simulink library "mbed_lib"  (R2016b)
settings: Solver=ode45  StartTime=0.0  StopTime=10.0  RelTol=1e-3
undefined symbols (not defined in the file): A, PortWidth
libraries: mbed_lib x1
settings Model: Creator=syoon  LastModifiedBy=oh
settings DataIOCC: LimitDataPoints=on  SaveFormat=Array
settings OptimizationCC: BlockReduction=off  BooleanDataType=off  LifeSpan=inf
settings DebuggingCC: SaveWithParameterizedLinksMsg=none  UnderspecifiedInitializationDetection=Classic  MergeDetectMultiDrivingBlocksExec=none  SignalResolutionControl=TryResolveAllWithWarning  StrictBusMsg=Warning  SFUnexpectedBacktrackingDiag=warning  SFNoUnconditionalDefaultTransitionDiag=warning  SFExecutionAtInitializationDiag=none
settings HardwareCC: ProdBitPerPointer=32  ProdBitPerSizeT=32  ProdBitPerPtrDiffT=32  ProdLargestAtomicFloat=None  ProdIntDivRoundTo=Undefined  ProdEndianess=Unspecified  ProdWordSize=32  ProdHWDeviceType=32-bit Generic  TargetUnknown=on
settings ModelReferenceCC: PropagateSignalLabelsOutOfModel=off
settings GRTTargetCC: TargetLangStandard=C89/C90 (ANSI)  GeneratePreprocessorConditionals=Disable all
settings ConfigComp: CovMetricSettings=dw  CovHtmlReporting=on  CovSaveCumulativeToWorkspaceVar=on  CovSaveSingleToWorkspaceVar=on  CovExternalEMLEnable=off  CovSFcnEnable=off

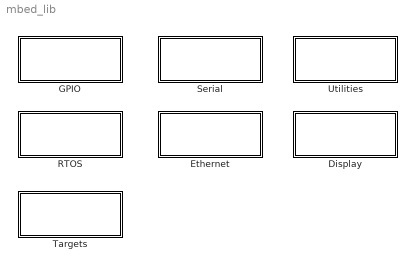
== system mbed_lib ==
  Display : Subsystem
      settings: OpenFcn=LCDScope
      mask Display: disp('Display')
  Ethernet : Subsystem
      settings: OpenFcn=mbed_ethernet
      mask Display: disp('Ethernet')
  GPIO : Subsystem
      mask Display: disp('GPIO')
  RTOS : Subsystem
      mask Display: disp('RTOS')
  Serial : Subsystem
      mask Display: disp('Serial')
  Targets : Subsystem
      settings: OpenFcn=mbed_targets
      mask Display: disp('Targets')
  Utilities : Subsystem
      mask Display: disp('Utilities')

== system mbed_lib/Display ==

== system mbed_lib/Ethernet ==

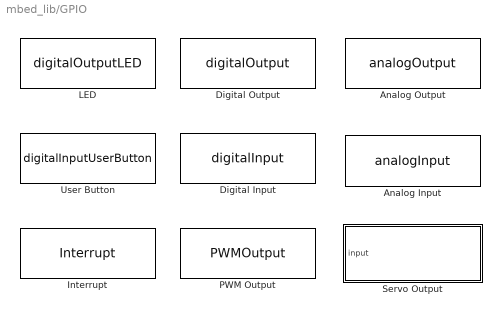
== system mbed_lib/GPIO ==
  Analog Input : S-Function  FunctionName=analogInput  Parameters=SampleTime, uint8(PortName), uint8(PinNumber)  SFunctionDeploymentMode=off  EnableBusSupport=off  mask(mbed Analog Input){PortName=A, PinNumber=0, SampleTime=-1}
      mask prompts: PortName "Port Name:"; PinNumber "Pin Number:"; SampleTime "Sample time (-1 for inherited):"
      mask help:
      | Reads the analog voltage input from the specified pin.
      |
      | The range of input on the pin is between 0 and Vref corresponding to a block output of 0 to 1.0f (in %) or 0 to 1024/4096/.. .
      mask Help: helpview(mbed_getHelpFile('analogInput'))
      mask TypeOptions PortName: A | B | C | D | E | F | G | H | I | J | K
      mask TypeOptions PinNumber: 0 | 1 | 2 | 3 | 4 | 5 | 6 | 7 | 8 | 9 | 10 | 11 | 12 | 13 | 14 | 15
      mask Display:
      | offset=0.0;
      | plot([0+offset:0.025:0.25+offset],0.3*sin(2*pi*[0:0.1:1])+0.5)
      | disp(['Pin ', PortName+64, '.', num2str(PinNumber-1)]);
      | port_label('output',1,'RAW');
      | port_label('output',2,'0-1.0f');
  Analog Output : S-Function  FunctionName=analogOutput  Parameters=SampleTime, uint8(PortName), uint8(PinNumber), uint8(Mode)  SFunctionDeploymentMode=off  EnableBusSupport=off  mask(mbed Analog Output){PortName=A, PinNumber=0, Mode=Double: 0 - 1.0f, SampleTime=-1}
      mask prompts: PortName "Port Name:"; PinNumber "Pin Number:"; Mode "Input data format"; SampleTime "Sample time (-1 for inherited):"
      mask help:
      | Writes an analog voltage output to the specified pin using the integrated DAC.
      |
      | The input to this block is a float between 0 and 1.0 (in %) or an integer between 0 and 1024/4096/.. corresponding to an output voltage between 0 to Vref.
      mask Help: helpview(mbed_getHelpFile('analogOutput'))
      mask TypeOptions PortName: A | B | C | D | E | F | G | H | I | J | K
      mask TypeOptions PinNumber: 0 | 1 | 2 | 3 | 4 | 5 | 6 | 7 | 8 | 9 | 10 | 11 | 12 | 13 | 14 | 15
      mask TypeOptions Mode: Uint16: RAW (0x0YYY) | Double: 0 - 1.0f
      mask Display:
      | offset=0.7;
      | plot([0+offset:0.025:0.25+offset],0.3*sin(2*pi*[0:0.1:1])+0.5)
      | disp(['Pin ', PortName+64, '.', num2str(PinNumber-1)]);
      | p={'RAW'; '0-1.0f'};
      | port_label('input',1,p{Mode});
  Digital Input : S-Function  FunctionName=digitalInput  Parameters=SampleTime, uint8(PortName), uint8(PinNumber), uint8(InputMode)  SFunctionDeploymentMode=off  EnableBusSupport=off  mask(mbed Digital Input){PortName=A, PinNumber=0, InputMode=PullDefault, SampleTime=-1}
      mask prompts: PortName "Port Name"; PinNumber "Pin Number:"; InputMode "Input Mode"; SampleTime "Sample time (-1 for inherited):"
      mask help:
      | Reads the digital value from the specified pin.
      |
      | The block outputs 1 for high and 0 for low.
      mask Help: helpview(mbed_getHelpFile('digitalInput'))
      mask TypeOptions PortName: A | B | C | D | E | F | G | H | I | J | K
      mask TypeOptions PinNumber: 0 | 1 | 2 | 3 | 4 | 5 | 6 | 7 | 8 | 9 | 10 | 11 | 12 | 13 | 14 | 15
      mask TypeOptions InputMode: PullDefault | PullUp | PullDown | PullNone
      mask Display:
      | plot([0 0.15 0.15 0.35 0.35 0.5],[0.3 0.3 0.7 0.7 0.3 0.3])
      | port_label('output',1,['Pin ', PortName+64, '.', num2str(PinNumber-1)]);
  Digital Output : S-Function  FunctionName=digitalOutput  Parameters=SampleTime, uint8(PortName), uint8(PinNumber), uint8(OutputMode)  SFunctionDeploymentMode=off  EnableBusSupport=off  mask(mbed Digital Output){PortName=A, PinNumber=0, OutputMode=PullDefault, SampleTime=-1}
      mask prompts: PortName "Port Name:"; PinNumber "Pin Number:"; OutputMode "Output Mode"; SampleTime "Sample time (-1 for inherited):"
      mask help:
      | Sends the digital value to the specified port.pin.
      |
      | The pin behaviour (pullup, pulldown, opendrain, ...) can be configured.
      |
      | An input of 1 sets the pin high and 0 sets the pin low.
      mask Help: helpview(mbed_getHelpFile('digitalOutput'))
      mask TypeOptions PortName: A | B | C | D | E | F | G | H | I | J | K
      mask TypeOptions PinNumber: 0 | 1 | 2 | 3 | 4 | 5 | 6 | 7 | 8 | 9 | 10 | 11 | 12 | 13 | 14 | 15
      mask TypeOptions OutputMode: PullDefault | PullUp | PullDown | PullNone | Repeater | OpenDrain
      mask Display:
      | plot([0.5 0.65 0.65 0.85 0.85 1],[0.3 0.3 0.7 0.7 0.3 0.3])
      | port_label('input',1,['Pin ', PortName+64, '.', num2str(PinNumber-1)]);
  Interrupt : S-Function  FunctionName=Interrupt  Parameters=uint8(PortName), uint8(PinNumber), uint8(Interrupt)  SFunctionDeploymentMode=off  EnableBusSupport=off  mask(mbed Interrupt Pin){PortName=A, PinNumber=0, Interrupt=Rise}
      mask prompts: PortName "Port Name"; PinNumber "Pin Name"
      mask help:
      | Defines the specified pin as an Interrupt pin. The interrupt can be generated by a rising, a falling or by both edges.
      |
      | A function-call subsystem can be connected with the output.
      mask Help: helpview(mbed_getHelpFile('Interrupt'))
      mask TypeOptions PortName: A | B | C | D | E | F | G | H | I | J | K
      mask TypeOptions PinNumber: 0 | 1 | 2 | 3 | 4 | 5 | 6 | 7 | 8 | 9 | 10 | 11 | 12 | 13 | 14 | 15
      mask TypeOptions Interrupt: None | Rise | Fall | Both
      mask Display:
      | p={'None'; 'Rise'; 'Fall'; 'Both'};
      | disp(['Interrupt: ' p{Interrupt} '          ']);
      | port_label('output',1,['Pin ', PortName+64, '.', num2str(PinNumber-1)]);
  LED : S-Function  FunctionName=digitalOutputLED  Parameters=SampleTime, uint8(nLED)  SFunctionDeploymentMode=off  EnableBusSupport=off  mask(mbed Digital Output LED){nLED=1, SampleTime=-1}
      mask prompts: nLED "LED Number:"; SampleTime "Sample time (-1 for inherited):"
      mask help:
      | Sends the digital value to the specified LED.
      |
      | An input of 1 sets the pin high and 0 sets the pin low.
      mask Help: helpview(mbed_getHelpFile('digitalOutputLED'))
      mask TypeOptions nLED: 1 | 2 | 3 | 4
      mask Display:
      | plot([0.5 0.65 0.65 0.85 0.85 0.85 1 0.5 0.65 0.65 0.85 0.85 0.85 1],[0.4 0.4 0.8 0.4 0.8 0.4 0.4 0.4 0.4 0.0 0.4 -0.0 0.4 0.4])
      | 
      | plot([0.75 0.8],[0.7 0.85])
      | plot([0.78 0.8],[0.825 0.85])
      | plot([0.79 0.8],[0.8 0.85])
      | 
      | plot([0.78 0.83],[0.7 0.85])
      | plot([0.815 0.83],[0.825 0.85])
      | plot([0.82 0.83],[0.8 0.85])
      | 
      | port_label('input',1,['LED' num2str(nLED)]);
  PWM Output : S-Function  FunctionName=PWMOutput  Parameters=SampleTime, uint8(PortName), uint8(PinNumber), uint32(Period)  SFunctionDeploymentMode=off  EnableBusSupport=off  mask(mbed PWM Output){PortName=A, PinNumber=0, Period=1000, SampleTime=-1}
      mask prompts: PortName "PWM Port:"; PinNumber "PWM Pin:"; Period "Period (µs):"; SampleTime "Sample time (-1 for inherited):"
      mask help:
      | Creates an pwm output signal on the specified pin using a configurable PWM period.
      |
      | The input to this block is a float between 0.0f and 1.0f corresponding to 0 to 100% pulsewidth.
      mask Help: helpview(mbed_getHelpFile('PWMOutput'))
      mask TypeOptions PortName: A | B | C | D | E | F | G | H | I | J | K
      mask TypeOptions PinNumber: 0 | 1 | 2 | 3 | 4 | 5 | 6 | 7 | 8 | 9 | 10 | 11 | 12 | 13 | 14 | 15
      mask Display:
      | plot([0.5 0.65 0.65 0.85 ],[0.3 0.3 0.7 0.7 ])
      | plot([0.8 0.8],[0.7 0.3])
      | plot([0.825 0.825],[0.7 0.3])
      | plot([0.85 0.85],[0.7 0.3])
      | plot([0.8 1],[0.3 0.3])
      | disp(['Pin ' PortName+64 '.' num2str(PinNumber-1)]);
      | port_label('input',1,'0-1.0f');
  Servo Output : Subsystem  mask(mbed Servo Output){PortName=A, PinNumber=0, PW_min=1, PW_max=2, SampleTime=-1}
      mask prompts: PortName "Port Name:"; PinNumber "Pin Number:"; PW_min "Pulse width min (ms)"; PW_max "max (ms)"; SampleTime "Sample time (-1 for inherited):"
      mask help:
      | Generates a PWM signal with a period of 20ms to control a standard RC-servo.
      | Minimal and maximal pulsewidth can be configured. Typical values are 1ms and 2ms.
      |
      | The input to this block is a float between 0.0f and 1.0f corresponding to a pulsewidth between the configured minimal to maximal values.
      mask Help: helpview(mbed_getHelpFile('Servo'))
      mask TypeOptions PortName: PWM Output/PortName
      mask TypeOptions PinNumber: PWM Output/PinNumber
      mask TypeOptions SampleTime: PWM Output/SampleTime
      mask Display:
      | disp('Servo Output\n');
      | disp(['\nPin ' PortName+64 '.' num2str(PinNumber-1) ]);
      | port_label('input',1,'0-1.0f');
  User Button : S-Function  FunctionName=digitalInputUserButton  Parameters=SampleTime  SFunctionDeploymentMode=off  EnableBusSupport=off  mask(mbed User Button){SampleTime=-1}
      mask prompts: SampleTime "Sample time (-1 for inherited):"
      mask help:
      | Reads the digital value from the User Button.
      |
      | The block outputs 1 for high and 0 for low. The
      mask Help: helpview(mbed_getHelpFile('digitalInputUserButton'))
      mask Display:
      | plot([0 0.15 0.35 ],[0.3 0.3 0.7])
      | plot([0.35 0.5],[0.3 0.3])
      | port_label('output',1,'UserButton');

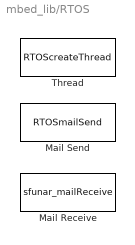
== system mbed_lib/RTOS ==
  Mail Receive : S-Function  FunctionName=sfunar_mailReceive  Parameters=MailNumber, uint32(DataType), uint32(NumElements)  SFunctionDeploymentMode=off  EnableBusSupport=off  mask{MailNumber=1, DataType=double, NumElements=1}
      mask prompts: MailNumber "Mail number"; DataType "Data type"; NumElements "Number of output elements"
      mask TypeOptions MailNumber: 1 | 2 | 3 | 4 | 5 | 6 | 7 | 8 | 9
      mask TypeOptions DataType: double | single | int8 | uint8 | int16 | uint16 | int32 | uint32
      mask Display:
      | disp(['Mail Receive\nInstance ' num2str(MailNumber)]);
      | port_label('output',1,'d');
      | port_label('output',2,'new');
  Mail Send : S-Function  FunctionName=RTOSmailSend  Parameters=MailNumber, DataType, uint32(NumElements), uint32(Depth)  SFunctionDeploymentMode=off  EnableBusSupport=off  mask(mbed RtosMail send){MailNumber=1, Depth=1, DataType=double, NumElements=1}
      mask prompts: MailNumber "Mail Instance Number"; Depth "Number of mails in queue"; DataType "Data type"; NumElements "Number of input elements"
      mask help:
      | Creates a rtos mailbox with the instance number 1...9.
      |
      | The maximal number of mails can be configured. Writing one mail more then this size will suspend the writing thread until the next mail is read.
      |
      | Each mail can contain the specified number of elements with the specified type.
      mask Help: helpview(mbed_getHelpFile('RTOSmailSend'))
      mask TypeOptions MailNumber: 1 | 2 | 3 | 4 | 5 | 6 | 7 | 8 | 9
      mask TypeOptions DataType: double | single | int8 | uint8 | int16 | uint16 | int32 | uint32
      mask Display:
      | disp(['Mail Send\nInstance ' num2str(MailNumber)]);
      | port_label('input',1,'d');
  Thread : S-Function  FunctionName=RTOScreateThread  Parameters=ThreadPriority, StackOption, uint32(StackSize), uint32(Timing)  SFunctionDeploymentMode=off  EnableBusSupport=off  mask(mbed create RTOS Thread){ThreadPriority=Normal, StackOption=Default, StackSize=0, Timing=0}
      mask prompts: ThreadPriority "Thread Priority"; StackOption "Stack size"; StackSize "Size: (bytes)"; Timing "Timing (ms)"
      mask help:
      | Creates a thread with the specified priority.
      |
      | Stack size can be DEFAULT_STACK_SIZE or have an individual value.
      |
      | When Timing equals 0, a Thread is created.
      | When Timing is greater then 0, a RtosTimer is created with this timing value (ms).
      | In both cases the function call subsystem is called in an endless loop (Thread) or a timed callback (RtosTimer).
      mask Help: helpview(mbed_getHelpFile('RTOScreateThread'))
      mask TypeOptions ThreadPriority: Idle | Low | Below Normal | Normal | Above Normal | High | Realtime
      mask TypeOptions StackOption: Default | User defined
      mask Display:
      | if Timing==0
      |   disp('create RtosThread');
      | else
      |   disp('create RtosTimer');
      | end

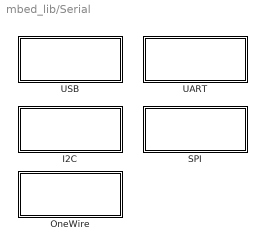
== system mbed_lib/Serial ==
  I2C : Subsystem
      mask Display: disp('I2C')
  OneWire : Subsystem
      mask Display: disp('OneWire')
  SPI : Subsystem
      mask Display: disp('SPI')
  UART : Subsystem
  USB : Subsystem

== system mbed_lib/Targets ==

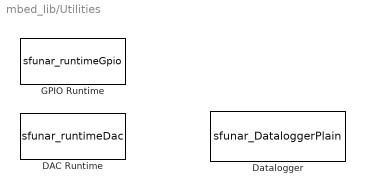
== system mbed_lib/Utilities ==
  DAC Runtime : S-Function  FunctionName=sfunar_runtimeDac  Parameters=SampleTime, PortName, PinNumber, DacValue  SFunctionDeploymentMode=off  EnableBusSupport=off  mask(DAC Runtime){PortName=A, PinNumber=0, DacValue=0, SampleTime=-1}
      mask prompts: PortName "Port Name"; PinNumber "Pin Number"; DacValue "DAC Value (0-1.0f)"; SampleTime "Sample time (-1 for inherited)"
      mask help:
      | Sets the DAC output to the configured value when entering the system that contains the block and resets the value after executing the systems code.
      | Can be used for time measurement of multiple subsystems, especially in multitasking models, using only one pin.
      | Setting each block to another DAC value and using an oscilloscope to differentiate between each subsystem.
      mask Help: helpview([mbed_getTargetRootPath '/doc/_build/htmlhelp/chapters/Dac_Runtime_en.html'])
      mask TypeOptions PortName: A | B | C | D | E | F | G | H | I | J
      mask TypeOptions PinNumber: 0 | 1 | 2 | 3 | 4 | 5 | 6 | 7 | 8 | 9 | 10 | 11 | 12 | 13 | 14 | 15
      mask Display:
      | disp('Runtime \nDAC Toggle\n');
      | disp(['\n\nPin ', PortName+64, '.', num2str(PinNumber-1) '  Value: ' num2str(DacValue) ]);
  Datalogger : S-Function  FunctionName=sfunar_DataloggerPlain  Parameters=TypeInputPorts, SampleTime, uint8(errEn), uint32(BufferSize)  SFunctionDeploymentMode=off  EnableBusSupport=off  mask(Creates a csv style string){TypeInputPorts={ 'uint8' 8 'int8' 4 'bool' 1 }, TypeOfInputs={'8*uint8' '4*int8' '1*bool'}, BufferSize=100, errEn=off, SampleTime=-1}
      mask prompts: TypeInputPorts "Type of Inputs"; TypeOfInputs "Type of Inputs"; BufferSize "Buffer Size"; errEn "Enable error output port"; SampleTime "Sample time (-1 for inherited):"
      mask help:
      | Type of Inputs:
      | List of 2-tuples
      |  1. item: Port width
      |  2. item: Port data type (single, double, int8, int16, int32, uint8, uint16, uint32, bool)
      |  e.g.: {'8*uint8' '4*int8' '1*bool'}
      |
      | Buffer Size:
      | Estimated maximal size of one data line.
      mask Callback TypeOfInputs:
      | cfg=eval(get_param(gcb,'TypeOfInputs'));
      | str={};
      | 
      | for i=1:size(cfg,2)
      |     res = strsplit(cfg{i}, '*');
      |     if isempty(str)
      |         str = strjoin({['''' res{2} ''''] res{1}});
      |     else
      |         str = strjoin({str ['''' res{2} ''''] res{1}});
      |     end
      | end
      | str = strjoin({'{' str '}'});
      | 
      | set_param(gcb,'TypeInputPorts', str);
      mask Display:
      | disp(['Datalogger']);
      | for i=1:2:size(TypeInputPorts,2)
      |     port_label('input',(i+1)/2, [TypeInputPorts{i} ':' num2str(TypeInputPorts{i+1})]);
      | end
      | port_label('output',1,'d');
      | port_label('output',2,'n');
      | if errEn
      |     port_label('output',3,'Error');
      | end
  GPIO Runtime : S-Function  FunctionName=sfunar_runtimeGpio  Parameters=SampleTime, PortName, PinNumber  SFunctionDeploymentMode=off  EnableBusSupport=off  mask(GPIO Runtime){PortName=A, PinNumber=0, SampleTime=-1}
      mask prompts: PortName "Port Name"; PinNumber "Pin Number"; SampleTime "Sample time (-1 for inherited)"
      mask help: Toggels a GPIO Pin so that the pulsewidth corresponds to the computational time of the containing subsystem.
      mask Help: helpview([mbed_getTargetRootPath '/doc/_build/htmlhelp/chapters/Gpio_Runtime_en.html'])
      mask TypeOptions PortName: A | B | C | D | E | F | G | H | I | J
      mask TypeOptions PinNumber: 0 | 1 | 2 | 3 | 4 | 5 | 6 | 7 | 8 | 9 | 10 | 11 | 12 | 13 | 14 | 15
      mask Display:
      | disp('Runtime \nGPIO Toggle\n');
      | disp(['\n\nPin ', PortName+64, '.', num2str(PinNumber-1)]);

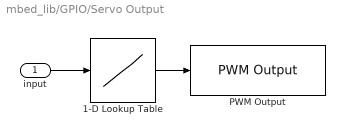
== system mbed_lib/GPIO/Servo Output ==
  input : Inport
  1-D Lookup Table : Lookup_n-D  NumberOfTableDimensions=1  BreakpointsForDimension1=[0 1]  Table=[PW_min PW_max]/20  ExtrapMethod=Clip  UseLastTableValue=on  InternalRulePriority=Speed  RndMeth=Simplest  InputSameDT=on
  PWM Output : mbed_lib/GPIO/PWM Output  PortName=A  PinNumber=0  Period=20000  SampleTime=SampleTime
  wires:
  input/1 -> 1-D Lookup Table/1
  1-D Lookup Table/1 -> PWM Output/1

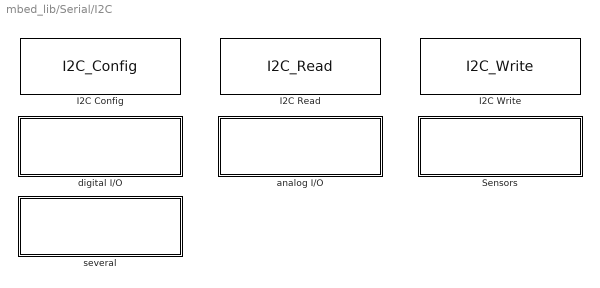
== system mbed_lib/Serial/I2C ==
  I2C Config : S-Function  Priority=0  FunctionName=I2C_Config  Parameters=uint8(SDAPortName), uint8(SDAPinNumber), uint8(SCLPortName), uint8(SCLPinNumber), uint32(Freq), uint8(I2CPort)  SFunctionDeploymentMode=off  EnableBusSupport=off  mask(I2C Configuration){I2CPort=1, Freq=100000, SDAPortName=B, SDAPinNumber=9, SCLPortName=B, SCLPinNumber=8}
      mask prompts: I2CPort "I2C Port"; Freq "Bus frequency: [Hz]"; SDAPortName "Port Name (SDA):"; SDAPinNumber "Pin Number:"; SCLPortName "Port Name (SCL):"; SCLPinNumber "Pin Number:"
      mask help:
      | This block sets up the I2C connection on the mbed board.
      |
      | To use several I2C busses at the mbed board, you can put several I2C Config blocks with different I2C Port numbers into the model. Each I2C Port number creates one instance of the mbed I2C class. The read and write blocks sending/receiving over the specific I2C bus have to use the same I2C Port number.
      mask Help: helpview(mbed_getHelpFile('I2CConfig'))
      mask TypeOptions I2CPort: 1 | 2 | 3
      mask TypeOptions SDAPortName: A | B | C | D | E | F
      mask TypeOptions SDAPinNumber: 0 | 1 | 2 | 3 | 4 | 5 | 6 | 7 | 8 | 9 | 10 | 11 | 12 | 13 | 14 | 15
      mask TypeOptions SCLPortName: A | B | C | D | E | F
      mask TypeOptions SCLPinNumber: 0 | 1 | 2 | 3 | 4 | 5 | 6 | 7 | 8 | 9 | 10 | 11 | 12 | 13 | 14 | 15
      mask Display:
      | disp(['I2C ' num2str(I2CPort) '\n\n']);
      | disp(['SDA: ' SDAPortName+64 '.' num2str(SDAPinNumber-1) ', SCL: ' SCLPortName+64, '.' num2str(SCLPinNumber-1)]);
      | disp(['\n\nFrequency: ' num2str(Freq) ' HZ']);
  I2C Read : S-Function  FunctionName=I2C_Read  Parameters=SampleTime, boolean(AddressFlag), uint8(SlaveAddress), boolean(ByteCountFlag), uint8(NumBytes), boolean(Repeated), uint8(I2cPort), boolean(AckOut)  SFunctionDeploymentMode=off  EnableBusSupport=off  mask(I2C Read){I2cPort=1, AddressFlag=off, SlaveAddress=0, ByteCountFlag=off, NumBytes=1, Repeated=off, AckOut=off, SampleTime=-1}
      mask prompts: I2cPort "I2C Port:"; AddressFlag "Enable address input port"; SlaveAddress "Slave address (8Bit):"; ByteCountFlag "Enable byte count input port"; NumBytes "Number of bytes to read:"; AckOut "Enable ack ouput port"; SampleTime "Sample time (-1 for inherited):"
      mask help: Performs a read operation from the device at the given i2c bus address.
      mask Help: helpview(mbed_getHelpFile('I2CRead'))
      mask TypeOptions I2cPort: 1 | 2 | 3
      mask Display:
      | disp(['I2C ' num2str(I2cPort) '\n']);
      | if AddressFlag == 0
      |     disp(['\nAddress: 0x' dec2hex(SlaveAddress)]);
      | else
      |    disp(['\nAddress: external']);
      |    port_label('input',1,'addr');
      | end
      | 
      | if ByteCountFlag == 1 && AddressFlag == 0
      |     port_label('input',1,'n');
      | elseif ByteCountFlag == 1 && AddressFlag == 1
      |     port_label('input',2,'n');
      | end
      | 
      | port_label('output',1,'d');
      | if AckOut == 1
      |     port_label('output',2,'ack');
      | end
  I2C Write : S-Function  FunctionName=I2C_Write  Parameters=SampleTime, boolean(AddressFlag), uint8(SlaveAddress), boolean(ByteCountFlag), boolean(Repeated), uint8(I2cPort), boolean(AckOut)  SFunctionDeploymentMode=off  EnableBusSupport=off  mask(I2C Write){I2cPort=1, AddressFlag=off, SlaveAddress=0, ByteCountFlag=off, Repeated=off, AckOut=off, SampleTime=-1}
      mask prompts: I2cPort "I2C Port:"; AddressFlag "Enable address input port"; SlaveAddress "Slave address (8Bit):"; ByteCountFlag "Enable byte count input port"; AckOut "Enable ack output port"; SampleTime "Sample time (-1 for inherited):"
      mask help: Performs a write operation to the device at the given i2c bus address.
      mask Help: helpview(mbed_getHelpFile('I2CWrite'))
      mask TypeOptions I2cPort: 1 | 2 | 3
      mask Display:
      | disp(['I2C ' num2str(I2cPort) '\n']);
      | 
      | port_label('input', 1, 'd');
      | 
      | if AddressFlag == 1
      |     disp(['\nAddress: external']);
      |     port_label('input', 2, 'addr');
      | else
      |     disp(['\nAddress: 0x' dec2hex(SlaveAddress)]);
      | end
      | 
      | if AddressFlag == 0 && ByteCountFlag == 1
      |     port_label('input', 2, 'n');
      | elseif AddressFlag == 1 && ByteCountFlag == 1
      |     port_label('input', 3, 'n');
      | end
      | 
      | if AckOut == 1
      |     port_label('output',1,'ack');
      | end
  Sensors : Subsystem
      settings: OpenFcn=mbed_i2c_sensors
  analog I/O : Subsystem
      settings: OpenFcn=mbed_i2c_analog_io
  digital I/O : Subsystem
      settings: OpenFcn=mbed_i2c_digital_io
  several : Subsystem
      settings: OpenFcn=mbed_i2c_several

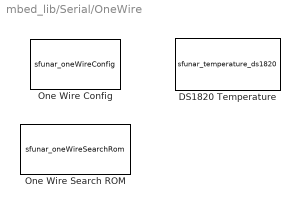
== system mbed_lib/Serial/OneWire ==
  DS1820 Temperature : S-Function  FunctionName=sfunar_temperature_ds1820  Parameters=OwBus, DeviceId, IDavail  SFunctionDeploymentMode=off  EnableBusSupport=off  mask(DS1820 Temperature){OwBus=1, DeviceId=[0 0 0 0 0 0]}
      mask prompts: OwBus "One Wire Bus"; DeviceId "Device ID (48 Bit)"
      mask help:
      | Reads the temperature measurement of a DS1820 (or DS18B20) One Wire temperature sensor.
      |
      | Output datatype:
      |     single
      mask init:
      | if (numel(DeviceId) == 0)
      |     IDavail = 0;
      |     DeviceId = 0;
      | else
      |     DeviceId = eval(DeviceId);
      |     if numel(DeviceId) ~= 6
      |         error('Device ID must contain 6 bytes');
      |     else
      |         IDavail = 1;
      |     end    
      | end
      mask Help: helpview([mbed_getTargetRootPath '/doc/_build/htmlhelp/sensor_actuator/DS1820_Temperature_en.html'])
      mask TypeOptions OwBus: 1 | 2 | 3 | 4 | 5 | 6 | 7 | 8 | 9
      mask Display:
      | disp(['DS1820 Temperature\n\n']);
      | disp(['\nOW Bus ' num2str(OwBus)]);
      | 
      | port_label('output',1,'°C');
  One Wire Config : S-Function  FunctionName=sfunar_oneWireConfig  Parameters=OwBus, OwPort, OwPin  SFunctionDeploymentMode=off  EnableBusSupport=off  mask(One Wire Config){OwBus=1, OwPort=A, OwPin=0}
      mask prompts: OwBus "OneWire Bus"; OwPort "OneWire Port:"; OwPin "Pin:"
      mask help: Configuration of a GPIO pin to be used as data line in a One Wire bus.
      mask Help: helpview([mbed_getTargetRootPath '/doc/_build/htmlhelp/mbed/one_wire_config_en.html'])
      mask TypeOptions OwBus: 1 | 2 | 3 | 4 | 5 | 6 | 7 | 8 | 9
      mask TypeOptions OwPort: A | B | C | D | E | F | G | H
      mask TypeOptions OwPin: 0 | 1 | 2 | 3 | 4 | 5 | 6 | 7 | 8 | 9 | 10 | 11 | 12 | 13 | 14 | 15
      mask Display:
      | disp('One Wire Config\n\n')
      | disp(['\nOW Bus ' num2str(OwBus)]);
      | disp(['\n\n\nPin: ' OwPort+64 '.' num2str(OwPin-1)]);
  One Wire Search ROM : S-Function  FunctionName=sfunar_oneWireSearchRom  Parameters=OwBus  SFunctionDeploymentMode=off  EnableBusSupport=off  mask{OwBus=1}
      mask prompts: OwBus "One Wire Bus"
      mask TypeOptions OwBus: 1 | 2 | 3 | 4 | 5 | 6 | 7 | 8 | 9
      mask Display:
      | disp('Search ROM\n\n')
      | disp(['\nOW Bus ' num2str(OwBus)]);
      | 
      | port_label('output',1,'ID');

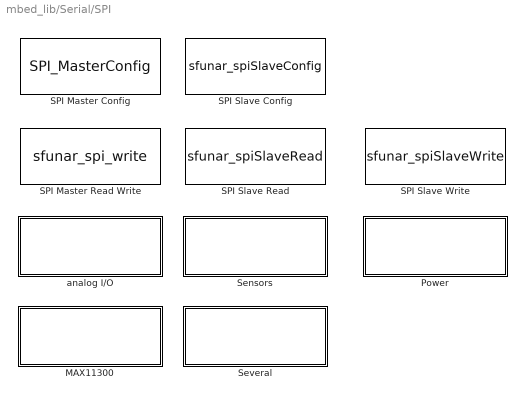
== system mbed_lib/Serial/SPI ==
  MAX11300 : Subsystem
      settings: OpenFcn=mbed_spi_max11300
  Power : Subsystem
      settings: OpenFcn=mbed_spi_power
  SPI Master Config : S-Function  Priority=0  FunctionName=SPI_MasterConfig  Parameters=uint8(MOSIPortName), uint8(MOSIPinNumber), uint8(MISOPortName), uint8(MISOPinNumber), uint8(SCLKPortName), uint8(SCLKPinNumber), uint32(Freq), uint8(Mode), uint8(Bits), uint8(SPIPort)  SFunctionDeploymentMode=off  EnableBusSupport=off  mask(SPI Configuration){SPIPort=1, Freq=100000, Mode=0, Bits=8, MOSIPortName=A, MOSIPinNumber=7, MISOPortName=A, MISOPinNumber=6, SCLKPortName=A, SCLKPinNumber=5}
      mask prompts: SPIPort "SPI Port"; Freq "Bus frequency: [Hz]"; MOSIPortName "MOSI: Port"; MOSIPinNumber "Pin"; MISOPortName "MISO: Port"; MISOPinNumber "Pin"; SCLKPortName "SCLK: Port"; SCLKPinNumber "Pin"
      mask help:
      | This block sets up the SPI connection on the mbed board. You must have one of these blocks in any model that ues SPI blocks.
      |
      | mode | POL PHA
      |  ------+--------
      |    0      |  0      0
      |    1      |  0      1
      |    2      |  1      0
      |    3      |  1      1
      mask Help: helpview([mbed_getTargetRootPath '/doc/_build/htmlhelp/chapters/Spi_Master_Config_en.html'])
      mask TypeOptions SPIPort: 1 | 2 | 3 | 4
      mask TypeOptions Mode: 0 | 1 | 2 | 3
      mask TypeOptions Bits: 4 | 5 | 6 | 7 | 8 | 9 | 10 | 11 | 12 | 13 | 14 | 15 | 16
      mask TypeOptions MOSIPortName: A | B | C | D | E | F | G | H | I | NC
      mask TypeOptions MOSIPinNumber: 0 | 1 | 2 | 3 | 4 | 5 | 6 | 7 | 8 | 9 | 10 | 11 | 12 | 13 | 14 | 15
      mask TypeOptions MISOPortName: A | B | C | D | E | F | G | H | I | NC
      mask TypeOptions MISOPinNumber: 0 | 1 | 2 | 3 | 4 | 5 | 6 | 7 | 8 | 9 | 10 | 11 | 12 | 13 | 14 | 15
      mask TypeOptions SCLKPortName: A | B | C | D | E | F | G | H | I
      mask TypeOptions SCLKPinNumber: 0 | 1 | 2 | 3 | 4 | 5 | 6 | 7 | 8 | 9 | 10 | 11 | 12 | 13 | 14 | 15
      mask Display:
      | disp(['SPI ' num2str(SPIPort) '\n\n\n']);
      | str1='';
      | if MOSIPortName==10
      |   str1 = 'NC';
      | else
      |   str1 = ['P' MOSIPortName+64 '.' num2str(MOSIPinNumber-1)];
      | end
      | str2='';
      | if MISOPortName==10
      |   str2 = 'NC';
      | else
      |   str2 = ['P' MISOPortName+64, '.' num2str(MISOPinNumber-1)];
      | end
      | disp(['\nMOSI: ' str1 ', MISO: ' str2 ' \n\n']);
      | disp(['\n\nSCK: P' SCLKPortName+64, '.' num2str(SCLKPinNumber-1) ' \n']);
      | disp(['\n\n\nFrequency: ' num2str(Freq) ' HZ']);
  SPI Master Read Write : S-Function  FunctionName=sfunar_spi_write  Parameters=SpiPort, CsPort, CsPin  SFunctionDeploymentMode=off  EnableBusSupport=off  mask(SPI Master Read Write){SpiPort=1, CsPort=A, CsPin=0}
      mask prompts: SpiPort "SPI Port"; CsPort "Chip Select Port"; CsPin "Pin"
      mask help: Perfoms a one byte write operation to the SPI bus and returns the received byte.
      mask Help: helpview([mbed_getTargetRootPath '/doc/_build/htmlhelp/chapters/Spi_Master_Read_Write_en.html'])
      mask TypeOptions SpiPort: 1 | 2 | 3 | 4
      mask TypeOptions CsPort: A | B | C | D | E | F | G | H
      mask TypeOptions CsPin: 0 | 1 | 2 | 3 | 4 | 5 | 6 | 7 | 8 | 9 | 10 | 11 | 12 | 13 | 14 | 15
      mask Display:
      | disp('SPI Master Read/Write\n\n');
      | disp(['SPI ' num2str(SpiPort)]);
      | 
      | disp(['\n\nChip Select: ' CsPort+64 '.' num2str(CsPin-1)]);
  SPI Slave Config : S-Function  FunctionName=sfunar_spiSlaveConfig  Parameters=BusSpeed, MosiPort, MosiPin, MisoPort, MisoPin, SckPort, SckPin, SselPort, SselPin  SFunctionDeploymentMode=off  EnableBusSupport=off  mask(SPI Slave Config){BusSpeed=100000, MosiPort=A, MosiPin=0, MisoPort=A, MisoPin=0, SckPort=A, SckPin=0, SselPort=A, SselPin=0}
      mask prompts: BusSpeed "Bus frequency: [Hz]"; MosiPort "MOSI: Port"; MosiPin "Pin"; MisoPort "MISO: Port"; MisoPin "Pin"; SckPort "SCK: Port"; SckPin "Pin"; SselPort "SSEL: Port"; SselPin "Pin"
      mask help: This block sets up the SPI connection on the mbed board to act as a slave device to an external master.
      mask Help: helpview([mbed_getTargetRootPath '/doc/_build/htmlhelp/chapters/Spi_Slave_Config_en.html'])
      mask TypeOptions MosiPort: A | B | C | D | E | F
      mask TypeOptions MosiPin: 0 | 1 | 2 | 3 | 4 | 5 | 6 | 7 | 8 | 9 | 10 | 11 | 12 | 13 | 14 | 15
      mask TypeOptions MisoPort: A | B | C | D | E | F
      mask TypeOptions MisoPin: 0 | 1 | 2 | 3 | 4 | 5 | 6 | 7 | 8 | 9 | 10 | 11 | 12 | 13 | 14 | 15
      mask TypeOptions SckPort: A | B | C | D | E | F
      mask TypeOptions SckPin: 0 | 1 | 2 | 3 | 4 | 5 | 6 | 7 | 8 | 9 | 10 | 11 | 12 | 13 | 14 | 15
      mask TypeOptions SselPort: A | B | C | D | E | F
      mask TypeOptions SselPin: 0 | 1 | 2 | 3 | 4 | 5 | 6 | 7 | 8 | 9 | 10 | 11 | 12 | 13 | 14 | 15
      mask Display:
      | disp(['Frequency: ' num2str(BusSpeed) ' HZ\n\n']);
      | disp(['\nMOSI: ' MosiPort+64 '.' num2str(MosiPin-1) ', MISO: ' MisoPort+64, '.' num2str(MisoPin-1) '\n']);
      | disp(['\n\n\nSCK: ' SckPort+64, '.' num2str(SckPin-1) ',SSEL: ' SselPort+64 '.' num2str(SselPin-1) '\n']);
  SPI Slave Read : S-Function  FunctionName=sfunar_spiSlaveRead  Parameters=SampleTime  SFunctionDeploymentMode=off  EnableBusSupport=off  mask(SPI Slave Read){SampleTime=-1}
      mask prompts: SampleTime "Sampel time: (-1 for inherited)"
      mask help: Reads the last received value from the spi input buffer.
      mask Help: helpview([mbed_getTargetRootPath '/doc/_build/htmlhelp/chapters/Spi_Slave_Read_en.html'])
      mask Display: disp('SPI Slave Read')
  SPI Slave Write : S-Function  FunctionName=sfunar_spiSlaveWrite  Parameters=SampleTime  SFunctionDeploymentMode=off  EnableBusSupport=off  mask(SPI Slave Write){SampleTime=-1}
      mask prompts: SampleTime "Sample time: (-1 for inherited)"
      mask help: This block puts one byte in the spi output buffer
      mask Help: helpview([mbed_getTargetRootPath '/doc/_build/htmlhelp/chapters/Spi_Slave_Write_en.html'])
      mask Display: disp('SPI Slave Write');
  Sensors : Subsystem
      settings: OpenFcn=mbed_spi_sensors
  Several : Subsystem
      settings: OpenFcn=mbed_spi_several
  analog I/O : Subsystem
      settings: OpenFcn=mbed_spi_analog_io

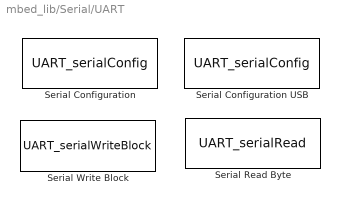
== system mbed_lib/Serial/UART ==
  Serial Configuration : S-Function  FunctionName=UART_serialConfig  Parameters=uint8(SerialPort), uint8(TXPort), uint8(TXPin), uint8(RXPort), uint8(RXPin), BaudRate  SFunctionDeploymentMode=off  EnableBusSupport=off  mask(mbed Serial Configuration){SerialPort=1, TXPort=A, TXPin=2, RXPort=A, RXPin=3, BaudRate=9600}
      mask prompts: SerialPort "Serial Port"; TXPort "Port Name (TX)"; TXPin "Pin Number (1-16):"; RXPort "Port Name (RX)"; RXPin "Pin Number (1-16):"; BaudRate "Baud Rate:"
      mask help:
      | This blocks sets up a serial connection on the mbed board. You must put at least one of these blocks into any model that ues the Serial Write or Serial Read blocks.
      |
      | To use several UARTS at the mbed board, you can put several Serial Config blocks with different Serial Port numbers into the model. Each Serial Port number creates one instance of the mbed Serial class. The read and write blocks sending/receiving over the specific UART have to use the same Serial Port number.
      |
      | Set the baud rate to match the device that you are communicating with. Standard rates include:300, 1200, 2400, 4800, 9600, 14400, 19200, 28800, 38400, 57600, or 115200.
      mask Help: helpview(mbed_getHelpFile('SerialUARTConfig'))
      mask TypeOptions SerialPort: 1 | 2 | 3 | 4 | 5
      mask TypeOptions TXPort: A | B | C | D | E | F
      mask TypeOptions TXPin: 0 | 1 | 2 | 3 | 4 | 5 | 6 | 7 | 8 | 9 | 10 | 11 | 12 | 13 | 14 | 15
      mask TypeOptions RXPort: A | B | C | D | E | F
      mask TypeOptions RXPin: 0 | 1 | 2 | 3 | 4 | 5 | 6 | 7 | 8 | 9 | 10 | 11 | 12 | 13 | 14 | 15
      mask Display: disp(['Serial config\nSerial' num2str(SerialPort) '\nTX ' TXPort+64 '.' num2str(TXPin-1) ', RX ' RXPort+64, '.' num2str(RXPin-1)]);
  Serial Configuration USB : S-Function  FunctionName=UART_serialConfig  Parameters=uint8(0), uint8(0), uint8(0), uint8(0), uint8(0), BaudRate  SFunctionDeploymentMode=off  EnableBusSupport=off  mask(mbed Serial Configuration){BaudRate=9600}
      mask prompts: BaudRate "Baud Rate:"
      mask help:
      | This blocks sets up the serial connection on the mbed board. You must have one of these blocks in any model that ues the Serial Write or Serial Read blocks.
      |
      | Set the baud rate to match the device that you are communicating with. Standard rates include:300, 1200, 2400, 4800, 9600, 14400, 19200, 28800, 38400, 57600, or 115200.
      mask Help: helpview(mbed_getHelpFile('SerialUARTConfigUSB'))
      mask Display: disp(['Serial config\nSerial0\nUSBTX, USBRX']);
  Serial Read Byte : S-Function  FunctionName=UART_serialRead  Parameters=SampleTime, uint8(SerialPort)  SFunctionDeploymentMode=off  EnableBusSupport=off  mask(mbed Serial Read){SerialPort=1, SampleTime=-1}
      mask prompts: SerialPort "Serial Port"; SampleTime "Sample time (-1 for inherited):"
      mask help:
      | Reads one byte from the serial port on the mbed board.
      |
      | Outputs -1 if no data is available to be read.
      mask Help: helpview(mbed_getHelpFile('SerialUARTRead'))
      mask TypeOptions SerialPort: 0 | 1 | 2 | 3 | 4 | 5
      mask Display:
      | p={'Serial0'; 'Serial1'; 'Serial2'; 'Serial3'; 'Serial4'; 'Serial5'};
      | disp(['Read Byte\n\n' p{SerialPort}])
  Serial Write Block : S-Function  FunctionName=UART_serialWriteBlock  Parameters=SampleTime, uint8(SerialPort), uint8(numData)  SFunctionDeploymentMode=off  EnableBusSupport=off  mask(mbed Serial Write){SerialPort=1, numData=on, SampleTime=-1}
      mask prompts: SerialPort "Serial Port"; numData "Enable datasize Port"; SampleTime "Sample time (-1 for inherited):"
      mask help: Writes the one dimensional vector of uint8 at input port d to the serial port on the mbed board. The length of the vector can be dynamically submitted at input port n or is statically read from input port d configuration.
      mask Help: helpview(mbed_getHelpFile('SerialUARTWriteBlock'))
      mask TypeOptions SerialPort: 0 | 1 | 2 | 3 | 4 | 5
      mask Display:
      | p={'Serial0'; 'Serial1'; 'Serial2'; 'Serial3'; 'Serial4'; 'Serial5'};
      | disp(['Write Block\n\n' p{SerialPort}])
      | port_label('input',1,'d');
      | if numData
      |     port_label('input',2,'n');
      | end

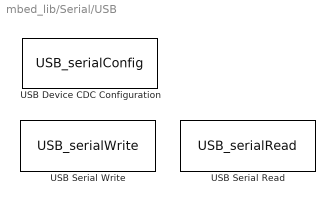
== system mbed_lib/Serial/USB ==
  USB Device CDC Configuration : S-Function  FunctionName=USB_serialConfig  SFunctionDeploymentMode=off  EnableBusSupport=off  mask(USB Device CDC (Virtual COM Port)){}
      mask help: This block sets up a virtual COM port via the native USB interface of the mcu.
      mask Help: helpview(mbed_getHelpFile('SerialUSBCDCConfig'))
      mask Display: disp(['USB Serial']);
  USB Serial Read : S-Function  FunctionName=USB_serialRead  Parameters=SampleTime, int32(PortWidth)  SFunctionDeploymentMode=off  EnableBusSupport=off  mask(mbed USB Serial Read){BufferSize=128, SampleTime=-1}
      mask prompts: BufferSize "Buffer Size"; SampleTime "Sample time (-1 for inherited):"
      mask help: Reads an vector of uint8 from USB CDC device driver and writes these data as an one dimensional vector to output port d. The length of the vector is min(Buffer Size, available data). At output port n the written vector size is available.
      mask Help: helpview(mbed_getHelpFile('SerialUSBCDCRead'))
      mask Display:
      | disp('USB Serial Read');
      | port_label('output',1,'d');
      | port_label('output',2,'n');
  USB Serial Write : S-Function  FunctionName=USB_serialWrite  Parameters=SampleTime, numData  SFunctionDeploymentMode=off  EnableBusSupport=off  mask(mbed USB Serial Write){numData=on, SampleTime=-1}
      mask prompts: numData "Enable datasize port"; SampleTime "Sample time (-1 for inherited):"
      mask help: Writes the one dimensional vector of uint8 at input port d to the USB CDC device driver. The length of the vector can be dynamically submitted at input port n or is statically read from input port d configuration.
      mask Help: helpview(mbed_getHelpFile('SerialUSBCDCWrite'))
      mask Display:
      | disp('USB Serial Write');
      | if numData == 1
      |     port_label('input',1,'d');
      |     port_label('input',2,'n');
      | end

== system mbed_lib/Serial/I2C/Sensors ==

== system mbed_lib/Serial/I2C/analog I//O ==

== system mbed_lib/Serial/I2C/digital I//O ==

== system mbed_lib/Serial/I2C/several ==

== system mbed_lib/Serial/SPI/MAX11300 ==

== system mbed_lib/Serial/SPI/Power ==

== system mbed_lib/Serial/SPI/Sensors ==

== system mbed_lib/Serial/SPI/Several ==

== system mbed_lib/Serial/SPI/analog I//O ==
